simulink model "ThreeTankRT"  (R2015b)
settings: Solver=ode5  SolverMode=SingleTasking  StartTime=0.0  StopTime=300  FixedStep=0.1  RelTol=1e-3
values from neighbouring files (symbols this model uses):
  H1 = [-33.648281245793970,3.333521763708310e+02]    [Initialise_MiniThreetank_System_C.m]    (also in LabScript.m; PolePlacementTest.m)
  H2 = [-33.765532144786600,3.358927606699081e+02]    [Initialise_MiniThreetank_System_C.m]    (also in LabScript.m; PolePlacementTest.m)
  H3 = [-33.660513524794340,3.290456571205451e+02]    [Initialise_MiniThreetank_System_C.m]    (also in LabScript.m; PolePlacementTest.m)
  P1 = [9.591077891437601,0.959107789143760]    [Initialise_MiniThreetank_System_C.m]    (also in LabScript.m; PolePlacementTest.m)
  P2 = [8.738131401544525,0.873813140154452]    [Initialise_MiniThreetank_System_C.m]    (also in LabScript.m; PolePlacementTest.m)
  Qlimit = 16    [Initialise_MiniThreetank_System_C.m]    (also in LabScript.m; PolePlacementTest.m)
undefined symbols (not defined in the file or in its folder): National_Instruments, PCIe
libraries: sldrtlib x2
settings Model: Creator=ksto036  LastModifiedBy=vsor436
settings DataIOCC: LimitDataPoints=off  SaveFormat=Array  SignalLoggingSaveFormat=ModelDataLogs  SaveOutput=off  SaveTime=off
settings OptimizationCC: ExpressionDepthLimit=2147483647
settings DebuggingCC: UnderspecifiedInitializationDetection=Classic  MergeDetectMultiDrivingBlocksExec=none  SolverPrmCheckMsg=warning  FcnCallInpInsideContextMsg=EnableAllAsWarning  UnconnectedInputMsg=none  UnconnectedOutputMsg=none  StateNameClashWarn=warning
settings HardwareCC: ProdBitPerPointer=32  ProdLargestAtomicFloat=None  ProdIntDivRoundTo=Undefined  ProdEndianess=Unspecified  ProdWordSize=32  ProdHWDeviceType=32-bit Generic
settings GRTTargetCC: GeneratePreprocessorConditionals=Disable all
settings ConfigComp: CovModelRefEnable=Off

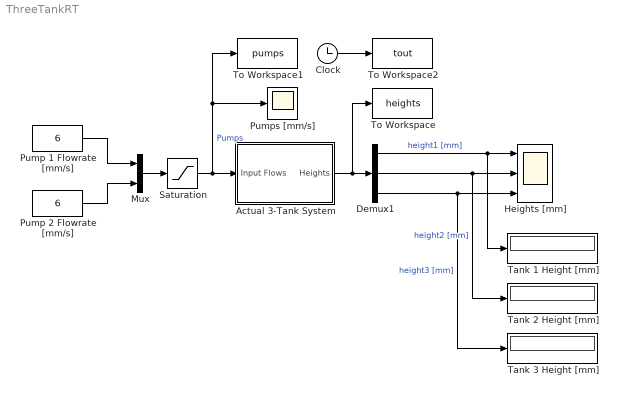
== system ThreeTankRT ==
  Actual 3-Tank System : Subsystem
  Clock : Clock
  Demux1 : Demux  Outputs=3
  Heights [mm] : Scope  NumInputPorts=3
  Mux : Mux  Inputs=2
  Pump 1 Flowrate [mm/s] : Constant  Value=6
  Pump 2 Flowrate [mm/s] : Constant  Value=6
  Pumps [mm/s] : Scope
  Saturation : Saturate  UpperLimit=Qlimit  LowerLimit=0  LinearizeAsGain=off
  Tank 1 Height [mm] : Display
  Tank 2 Height [mm] : Display
  Tank 3 Height [mm] : Display
  To Workspace : ToWorkspace  VariableName=heights  SampleTime=-1
  To Workspace1 : ToWorkspace  VariableName=pumps  SampleTime=-1
  To Workspace2 : ToWorkspace  VariableName=tout  SampleTime=-1
  wires:
  Mux/1 -> Saturation/1
  Pump 1 Flowrate [mm/s]/1 -> Mux/1
  Pump 2 Flowrate [mm/s]/1 -> Mux/2
  Actual 3-Tank System/1(Heights) -> To Workspace/1, Demux1/1
  Demux1/3 -> Tank 3 Height [mm]/1, Heights [mm]/3  "height3 [mm]"
  Demux1/2 -> Tank 2 Height [mm]/1, Heights [mm]/2  "height2 [mm]"
  Demux1/1 -> Tank 1 Height [mm]/1, Heights [mm]/1  "height1 [mm]"
  Saturation/1 -> Pumps [mm/s]/1, To Workspace1/1, Actual 3-Tank System/1(Input Flows)  "Pumps"
  Clock/1 -> To Workspace2/1

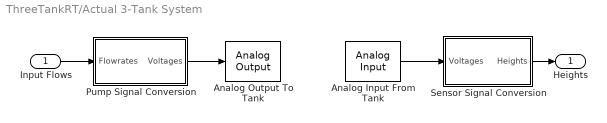
== system ThreeTankRT/Actual 3-Tank System ==
  Input Flows : Inport
  Analog Input From Tank : sldrtlib/Analog Input  SampleTime=0.1  MaxMissedTicks=10  ShowMissedTicks=off  YieldWhenWaiting=off  DrvName=National_Instruments/PCIe-6321  DrvAddress=4294967295  DrvOptions=[0 0 0 0 0 0 0]  Channels=[1 2 3]  RangeMode=1  VoltRange=1  DataType=1
      settings: AttributesFormatString=National Instruments\nPCIe-6321 [auto]
  Analog Output To Tank : sldrtlib/Analog Output  SampleTime=0.1  MaxMissedTicks=10  ShowMissedTicks=off  YieldWhenWaiting=off  DrvName=National_Instruments/PCIe-6321  DrvAddress=4294967295  DrvOptions=[0 0 0 0 0 0 0]  Channels=[1 2]  RangeMode=1  VoltRange=1  InitialValue=[-10]  FinalValue=[-10]
      settings: AttributesFormatString=National Instruments\nPCIe-6321 [auto]
  Pump Signal Conversion : Subsystem
  "Sensor Signal Conversion " : Subsystem
  Heights : Outport
  wires:
  Pump Signal Conversion/1(Voltages) -> Analog Output To Tank/1
  Analog Input From Tank/1 -> "Sensor Signal Conversion "/1(Voltages)
  Input Flows/1 -> Pump Signal Conversion/1(Flowrates)
  "Sensor Signal Conversion "/1(Heights) -> Heights/1

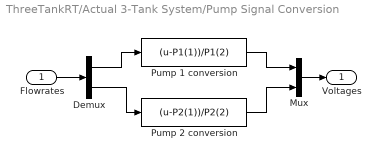
== system ThreeTankRT/Actual 3-Tank System/Pump Signal Conversion ==
  Flowrates : Inport
  Demux : Demux  Outputs=2
  Mux : Mux  Inputs=2
  Pump 1 conversion : Fcn  Expr=(u-P1(1))/P1(2)
  Pump 2 conversion : Fcn  Expr=(u-P2(1))/P2(2)
  Voltages : Outport
  wires:
  Mux/1 -> Voltages/1
  Pump 1 conversion/1 -> Mux/1
  Pump 2 conversion/1 -> Mux/2
  Flowrates/1 -> Demux/1
  Demux/1 -> Pump 1 conversion/1
  Demux/2 -> Pump 2 conversion/1

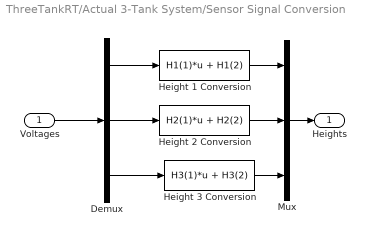
== system ThreeTankRT/Actual 3-Tank System/Sensor Signal Conversion  ==
  Voltages : Inport
  Demux : Demux  Outputs=3
  Height 1 Conversion : Fcn  Expr=H1(1)*u + H1(2)
  Height 2 Conversion : Fcn  Expr=H2(1)*u + H2(2)
  Height 3 Conversion : Fcn  Expr=H3(1)*u + H3(2)
  Mux : Mux  Inputs=3
  Heights : Outport
  wires:
  Voltages/1 -> Demux/1
  Demux/1 -> Height 1 Conversion/1
  Demux/2 -> Height 2 Conversion/1
  Demux/3 -> Height 3 Conversion/1
  Height 1 Conversion/1 -> Mux/1
  Height 2 Conversion/1 -> Mux/2
  Height 3 Conversion/1 -> Mux/3
  Mux/1 -> Heights/1
